simulink model "AttitudeSimulation"  (R2019a)
settings: Solver=VariableStepAuto  StartTime=0.0  StopTime=999  FixedStep=0.01  RelTol=1e-3
libraries: vrlib x1
settings Model: Creator=user  LastModifiedBy=Cal__
settings DataIOCC: ReturnWorkspaceOutputs=off
settings DebuggingCC: ArithmeticOperatorsInVariantConditions=warning

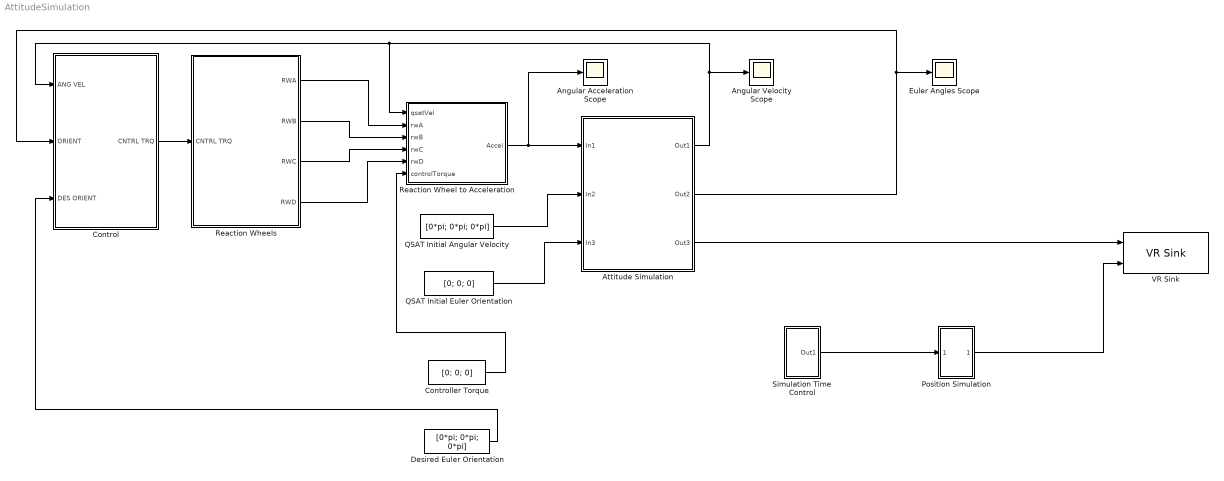
== system AttitudeSimulation ==
  Angular Acceleration Scope : Scope
  Angular Velocity Scope : Scope
  Attitude Simulation : Subsystem
  Control : Subsystem
  Controller Torque : Constant  Value=[0; 0; 0]
  Desired Euler Orientation : Constant  Value=[0*pi; 0*pi; 0*pi]
  Euler Angles Scope : Scope
  Position Simulation : Subsystem
  QSAT Initial Angular Velocity : Constant  Value=[0*pi; 0*pi; 0*pi]
  QSAT Initial Euler Orientation : Constant  Value=[0; 0; 0]
  Reaction Wheel to Acceleration : MATLAB Function  TreatAsAtomicUnit=on
  Reaction Wheels : Subsystem
  Simulation Time Control : Subsystem
  VR Sink : vrlib/VR Sink  InstantiateOnLoad=on  SampleTime=0.1  ViewEnable=on  RemoteChange=off  RemoteView=off  FieldsWritten=STLB_transform.rotation.4.1.1.double#STLB_transform.translation.3.1.1.double  WorldFileName=world.wrl  AutoView=on  VideoDimensions=[]  AllowVariableSize=off
      settings: SourceProductBaseCode=VR
  wires:
  Reaction Wheel to Acceleration/1(Accel) -> Attitude Simulation/1(In1), Angular Acceleration Scope/1
  Controller Torque/1 -> Reaction Wheel to Acceleration/6(controlTorque)
  Reaction Wheels/1(RWA) -> Reaction Wheel to Acceleration/2(rwA)
  Reaction Wheels/2(RWB) -> Reaction Wheel to Acceleration/3(rwB)
  Reaction Wheels/3(RWC) -> Reaction Wheel to Acceleration/4(rwC)
  Reaction Wheels/4(RWD) -> Reaction Wheel to Acceleration/5(rwD)
  Desired Euler Orientation/1 -> Control/3(DES ORIENT)
  Control/1(CNTRL TRQ) -> Reaction Wheels/1(CNTRL TRQ)
  Simulation Time Control/1(Out1) -> Position Simulation/1(In1)
  Position Simulation/1(Out1) -> VR Sink/2
  Attitude Simulation/2(Out2) -> Control/2(ORIENT), Euler Angles Scope/1
  Attitude Simulation/1(Out1) -> Control/1(ANG VEL), Reaction Wheel to Acceleration/1(qsatVel), Angular Velocity Scope/1
  QSAT Initial Angular Velocity/1 -> Attitude Simulation/2(In2)
  QSAT Initial Euler Orientation/1 -> Attitude Simulation/3(In3)
  Attitude Simulation/3(Out3) -> VR Sink/1

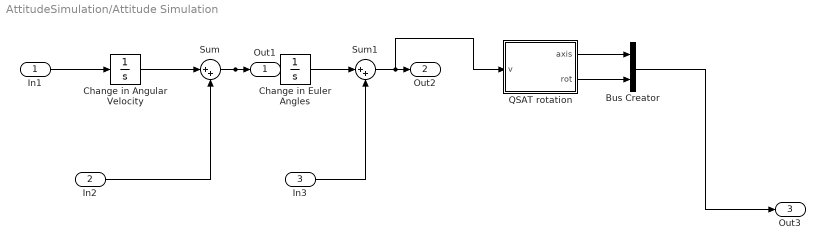
== system AttitudeSimulation/Attitude Simulation ==
  In1 : Inport
  In2 : Inport  Port=2
  In3 : Inport  Port=3
  Bus Creator : BusCreator  Inputs=2
  Change in Angular Velocity : Integrator
  Change in Euler Angles : Integrator
  QSAT rotation : MATLAB Function  TreatAsAtomicUnit=on
  Sum : Sum  Inputs=|++
  Sum1 : Sum  Inputs=|++
  Out1 : Outport
  Out2 : Outport  Port=2
  Out3 : Outport  Port=3
  wires:
  QSAT rotation/2(rot) -> Bus Creator/2
  In1/1 -> Change in Angular Velocity/1
  In3/1 -> Sum1/2
  Change in Euler Angles/1 -> Sum1/1
  Sum/1 -> Change in Euler Angles/1, Out1/1
  Change in Angular Velocity/1 -> Sum/1
  QSAT rotation/1(axis) -> Bus Creator/1
  In2/1 -> Sum/2
  Sum1/1 -> QSAT rotation/1(v), Out2/1
  Bus Creator/1 -> Out3/1

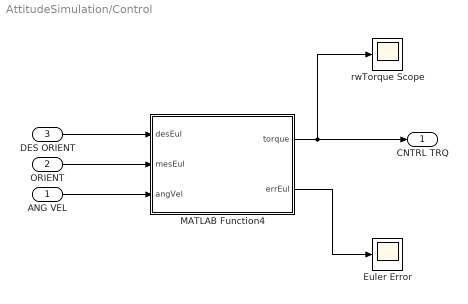
== system AttitudeSimulation/Control ==
  ANG VEL : Inport
  ORIENT : Inport  Port=2
  DES ORIENT : Inport  Port=3
  Euler Error : Scope
  MATLAB Function4 : MATLAB Function  TreatAsAtomicUnit=on
  rwTorque Scope : Scope
  CNTRL TRQ : Outport
  wires:
  ANG VEL/1 -> MATLAB Function4/3(angVel)
  MATLAB Function4/1(torque) -> CNTRL TRQ/1, rwTorque Scope/1
  MATLAB Function4/2(errEul) -> Euler Error/1
  DES ORIENT/1 -> MATLAB Function4/1(desEul)
  ORIENT/1 -> MATLAB Function4/2(mesEul)

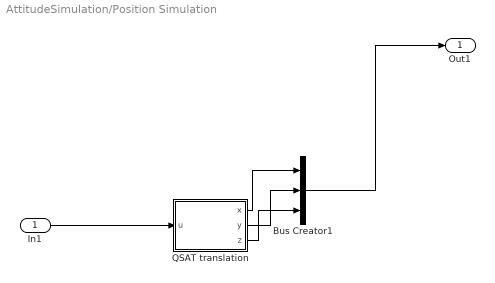
== system AttitudeSimulation/Position Simulation ==
  In1 : Inport
  Bus Creator1 : BusCreator  Inputs=3
  "QSAT translation " : MATLAB Function  TreatAsAtomicUnit=on
  Out1 : Outport
  wires:
  In1/1 -> "QSAT translation "/1(u)
  "QSAT translation "/1(x) -> Bus Creator1/1
  "QSAT translation "/2(y) -> Bus Creator1/2
  "QSAT translation "/3(z) -> Bus Creator1/3
  Bus Creator1/1 -> Out1/1

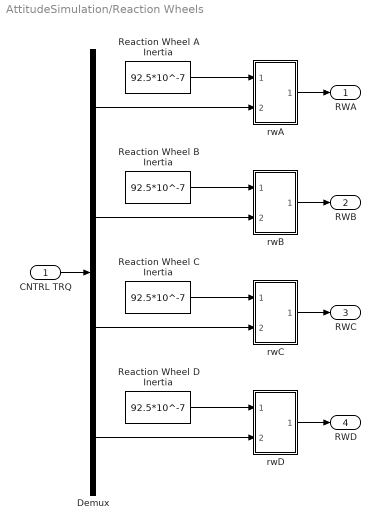
== system AttitudeSimulation/Reaction Wheels ==
  CNTRL TRQ : Inport
  Demux : Demux
  Reaction Wheel A Inertia : Constant  Value=92.5*10^-7
  Reaction Wheel B Inertia : Constant  Value=92.5*10^-7
  Reaction Wheel C Inertia : Constant  Value=92.5*10^-7
  Reaction Wheel D Inertia : Constant  Value=92.5*10^-7
  rwA : Subsystem
  rwB : Subsystem
  rwC : Subsystem
  rwD : Subsystem
  RWA : Outport
  RWB : Outport  Port=2
  RWC : Outport  Port=3
  RWD : Outport  Port=4
  wires:
  Demux/2 -> rwB/2(In2)
  Reaction Wheel C Inertia/1 -> rwC/1(In1)
  Demux/4 -> rwD/2(In2)
  Reaction Wheel A Inertia/1 -> rwA/1(In1)
  Demux/3 -> rwC/2(In2)
  Demux/1 -> rwA/2(In2)
  Reaction Wheel D Inertia/1 -> rwD/1(In1)
  Reaction Wheel B Inertia/1 -> rwB/1(In1)
  CNTRL TRQ/1 -> Demux/1
  rwC/1(rwC) -> RWC/1
  rwD/1(rwD) -> RWD/1
  rwB/1(rwB) -> RWB/1
  rwA/1(rwA) -> RWA/1

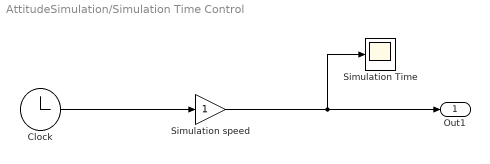
== system AttitudeSimulation/Simulation Time Control ==
  "Clock " : Clock
  "Simulation Time " : Scope
  Simulation speed : Gain
  Out1 : Outport
  wires:
  "Clock "/1 -> Simulation speed/1
  Simulation speed/1 -> Out1/1, "Simulation Time "/1

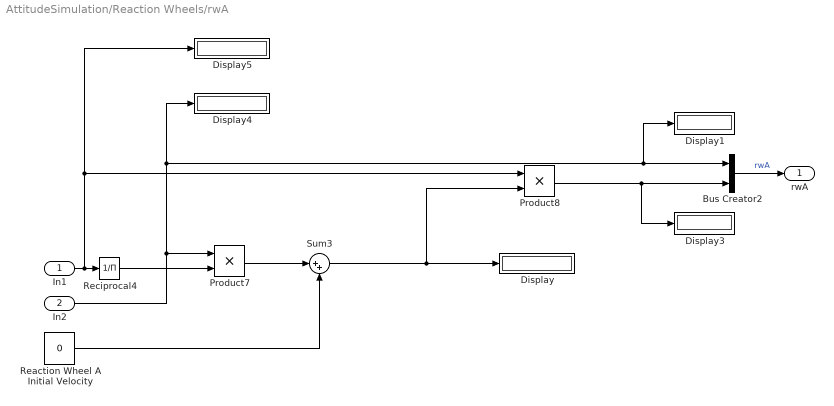
== system AttitudeSimulation/Reaction Wheels/rwA ==
  In1 : Inport
  In2 : Inport  Port=2
  Bus Creator2 : BusCreator  Inputs=2
  Display{,1,3..5} (5 alike) : Display
  Product7 : Product
  Product8 : Product
  Reaction Wheel A Initial Velocity : Constant  Value=0
  Reciprocal4 : Product  Inputs=/
  Sum3 : Sum  Inputs=|++
  rwA : Outport
  wires:
  In2/1 -> Display4/1, Display1/1, Bus Creator2/1, Product7/1
  Product7/1 -> Sum3/1
  Product8/1 -> Display3/1, Bus Creator2/2
  Sum3/1 -> Product8/2, Display/1
  In1/1 -> Display5/1, Product8/1, Reciprocal4/1
  Bus Creator2/1 -> rwA/1  "rwA"
  Reciprocal4/1 -> Product7/2
  Reaction Wheel A Initial Velocity/1 -> Sum3/2

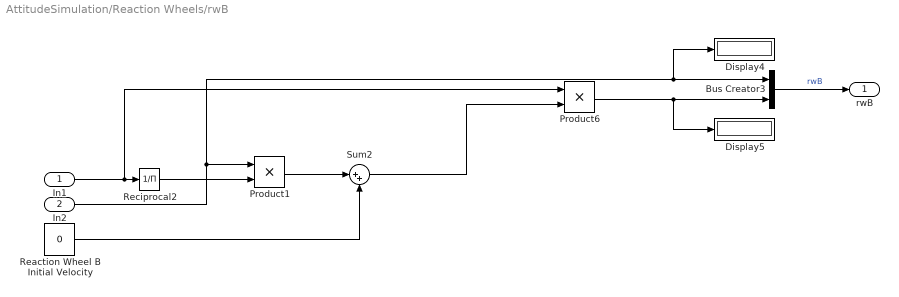
== system AttitudeSimulation/Reaction Wheels/rwB ==
  In1 : Inport
  In2 : Inport  Port=2
  Bus Creator3 : BusCreator  Inputs=2
  Display4 : Display
  Display5 : Display
  Product1 : Product
  Product6 : Product
  Reaction Wheel B Initial Velocity : Constant  Value=0
  Reciprocal2 : Product  Inputs=/
  Sum2 : Sum  Inputs=|++
  rwB : Outport
  wires:
  Reciprocal2/1 -> Product1/2
  In2/1 -> Display4/1, Bus Creator3/1, Product1/1
  Reaction Wheel B Initial Velocity/1 -> Sum2/2
  In1/1 -> Product6/1, Reciprocal2/1
  Product6/1 -> Display5/1, Bus Creator3/2
  Product1/1 -> Sum2/1
  Bus Creator3/1 -> rwB/1  "rwB"
  Sum2/1 -> Product6/2

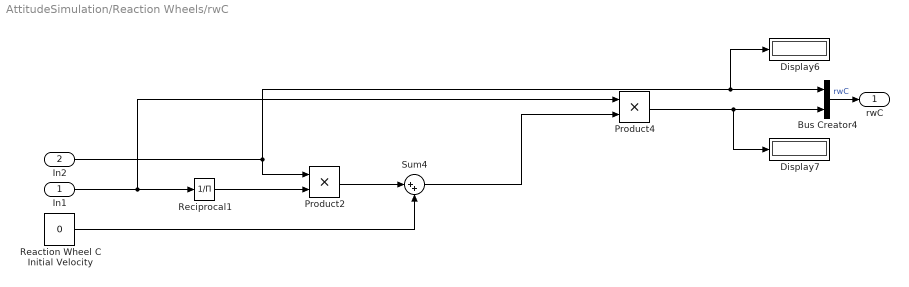
== system AttitudeSimulation/Reaction Wheels/rwC ==
  In1 : Inport
  In2 : Inport  Port=2
  Bus Creator4 : BusCreator  Inputs=2
  Display6 : Display
  Display7 : Display
  Product2 : Product
  Product4 : Product
  Reaction Wheel C Initial Velocity : Constant  Value=0
  Reciprocal1 : Product  Inputs=/
  Sum4 : Sum  Inputs=|++
  rwC : Outport
  wires:
  Product4/1 -> Display7/1, Bus Creator4/2
  Product2/1 -> Sum4/1
  Reciprocal1/1 -> Product2/2
  Reaction Wheel C Initial Velocity/1 -> Sum4/2
  Bus Creator4/1 -> rwC/1  "rwC"
  In2/1 -> Display6/1, Bus Creator4/1, Product2/1
  In1/1 -> Product4/1, Reciprocal1/1
  Sum4/1 -> Product4/2

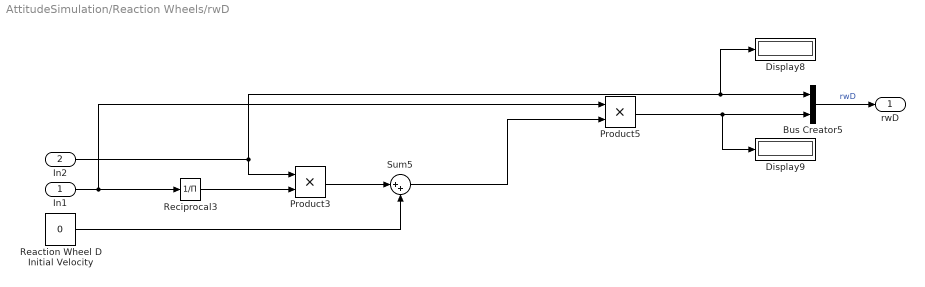
== system AttitudeSimulation/Reaction Wheels/rwD ==
  In1 : Inport
  In2 : Inport  Port=2
  Bus Creator5 : BusCreator  Inputs=2
  Display8 : Display
  Display9 : Display
  Product3 : Product
  Product5 : Product
  Reaction Wheel D Initial Velocity : Constant  Value=0
  Reciprocal3 : Product  Inputs=/
  Sum5 : Sum  Inputs=|++
  rwD : Outport
  wires:
  Product3/1 -> Sum5/1
  Reciprocal3/1 -> Product3/2
  Product5/1 -> Display9/1, Bus Creator5/2
  Reaction Wheel D Initial Velocity/1 -> Sum5/2
  Bus Creator5/1 -> rwD/1  "rwD"
  In2/1 -> Display8/1, Bus Creator5/1, Product3/1
  In1/1 -> Product5/1, Reciprocal3/1
  Sum5/1 -> Product5/2

== matlab function AttitudeSimulation/Position Simulation/QSAT translation  ==
  data: x output; u input; y output; z output
function [x,y,z] = fcn(u)
    x=0;
    y=0;
    z=0;
end

== matlab function AttitudeSimulation/Attitude Simulation/QSAT rotation ==
  data: axis output; v input; rot output
function [axis,rot] = fcn(v)
    
    %setup for manipulation
    cx = cos(v(1)/2);
    cy = cos(v(2)/2);
    cz = cos(v(3)/2);
    
    sx = sin(v(1)/2);
    sy = sin(v(2)/2);
    sz = sin(v(3)/2);
    
    %axis calculation
    x = sx*sy*cz + cx*cy*sz;
    y = sx*cy*cz + cx*sy*sz;
    z = cx*sy*cz - sx*cy*sz;
    
    axis = [x, y, z];
    
    %magnitude calculation
    rot = 2*acos(cx*cy*cz - sx*sy*sz);
end

== matlab function AttitudeSimulation/Reaction Wheel to Acceleration ==
  data: qsatVel input; rwA input; rwB input; rwC input; rwD input; controlTorque input; Accel output
function Accel = fcn(qsatVel, rwA, rwB, rwC, rwD,controlTorque)
%where each rw is a vector containing momentum and torque along the wheel's axis (elevation assumed to be pi/4)
    %rwA is on x
    %rwB is on y
    %rwC is on -x
    %rwD is on -y
    
%find ReactionWheel momentum and torque with respect to cubeSat coordinates
    a = cos(pi/4); %as cos(pi/4) == sin(pi/4)
    x = [0,0];
    y = [0,0];
    z = [0,0];
    for i = 1 : 2
        x(i) = a*(rwA(i) - rwC(i));
        y(i) = a*(rwB(i) - rwD(i));
        z(i) = a*(rwA(i) + rwB(i) + rwC(i) + rwD(i));
    end
    rwMomentum = [x(1); y(1); z(1)];
    rwTorque = [x(2); y(2); z(2)];
    
%find acceleration due to controller, reaction wheel, and cubeSat properties
    qsatInertia = [0.03480965677, -0.00003570019, -0.00070790838;
                  -0.00003570019,  0.03272823537, -0.00002125943;
                  -0.00070790838, -0.00002125943,  0.00876862587];
    qsatVelocity = qsatVel;
    %manipulation for equation
    invI = inv(qsatInertia);
    crossVel = [             0, -qsatVelocity(3), qsatVelocity(2);
               qsatVelocity(3),                0,-qsatVelocity(1);
              -qsatVelocity(2),  qsatVelocity(1),              0];            
    Hw = rwMomentum;
    Tw = rwTorque;
    Tc = controlTorque;
    %acceleration equation      
    Accel = -invI*crossVel*qsatInertia*qsatVelocity-invI*crossVel*Hw-invI*Tw-invI*Tc;

== matlab function AttitudeSimulation/Control/MATLAB Function4 ==
  data: desEul input; torque output; mesEul input; errEul output; angVel input
function [torque, errEul] = RotationConversion(desEul, mesEul, angVel)

    angVelEul = angVel*20;
    %placeholder for integral
    
    mesEul = mod(mesEul, [2*pi;2*pi;2*pi]);
    for i = 1 : 3
        if mesEul(i) > 1.25*pi
            mesEul(i) = mesEul(i) - 2*pi;
        elseif mesEul(i) < -1.25*pi
            mesEul(i) = mesEul(i) + 2*pi;
        end
    end
    %removes extra rotations based on previous turns
    
    errEul = -.1*(desEul - mesEul - angVelEul);
    
    errWA = errEul(1);
    errWB = (errEul(3) - errEul(1) + errEul(2))/2;
    errWC = 0;
    errWD = errWB - errEul(2);
    %only 3 reaction wheels are needed
    temp = [errWA, errWB, errWC, errWD];
     
    mult = 1;
    for i = 1 : 4
        if temp(i) > 0.05
            mult = temp(i)/0.05;
        end
    end
    
    temp = temp./mult;
    
    %max torque is 50mNm or 0.050Nm
    torque = temp;
    
end
